simulink model "chain"  (R2022a)
settings: Solver=VariableStepAuto  StartTime=0.0  StopTime=1000  RelTol=1e-3
undefined symbols (not defined in the file): None, S, vsva2197, xcvc1902
libraries: aieBasic x4, aieUtilities x3, dspmlti4 x2, aieDSP x2, hdlUtilities x2, dspsrcs4 x1, vmcUtilities x1, hdlDSPIP x1
settings Model: Creator=abehbood  LastModifiedBy=abehbood
settings ModelReferenceCC: EnableRefExpFcnMdlSchedulingChecks=off
settings RTWCC: Description=Generic Real-Time Target

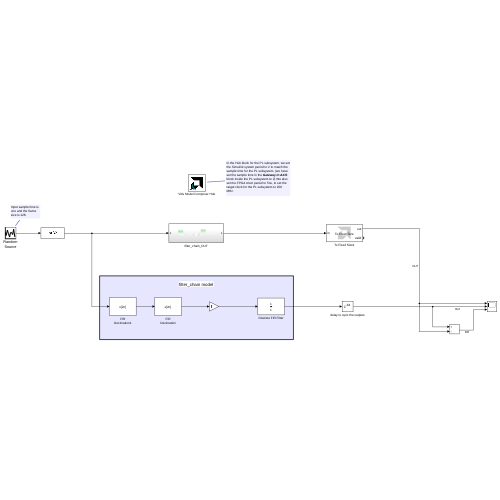
[thumbnail: Simulink's stored preview of the top-level diagram]
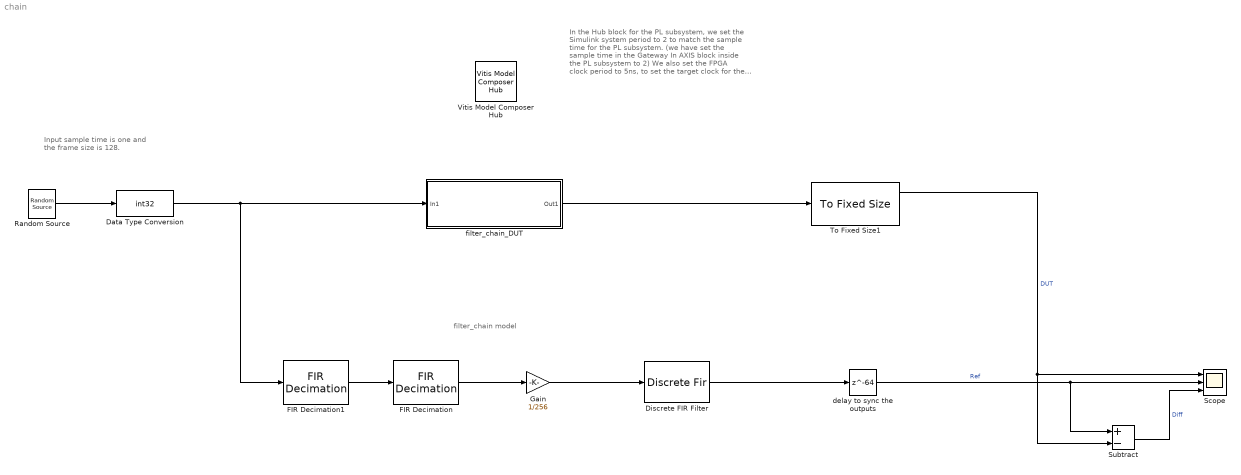
== system chain ==
  note: In the Hub block for the PL subsystem, we set the Simulink system period to 2 to match the sample time for the PL subsystem. (we have set the sample time in the Gateway In AXIS block inside the PL subsystem to 2) We also set the FPGA clock period to 5ns, to set the target clock for the PL subsystem to 200 MHz.
  note: filter_chain model
  note: Input sample time is one and the frame size is 128.
  Data Type Conversion : DataTypeConversion  OutDataTypeStr=int32  SaturateOnIntegerOverflow=off  RndMeth=Floor
  Discrete FIR Filter : DiscreteFir  Coefficients=1  InputProcessing=Columns as channels (frame based)  OutDataTypeStr=Inherit: Same as input
  FIR Decimation : dspmlti4/FIR Decimation  FilterSource=Dialog parameters  h=[6,0,-4,-3,5,6,-6,-13,7,44,64,44,7,-13,-6,6,5,-3,-4,0,6]  D=2  filtStruct=Direct form  FilterObject=FDECIM  InputProcessing=Columns as channels (frame based)  framing=Enforce single-rate processing  inputOffset=0  outputBufInitCond=0  roundingMode=Floor  overflowMode=off  firstCoeffDataTypeStr=Inherit: Same word length as input  firstCoeffMin=[]  firstCoeffMax=[]  firstCoeffLastDataTypeStr=Inherit: Same word length as input  outputMin=[]  outputMax=[]
  FIR Decimation1 : dspmlti4/FIR Decimation  FilterSource=Dialog parameters  h=1  D=2  filtStruct=Direct form  FilterObject=FDECIM  InputProcessing=Columns as channels (frame based)  framing=Enforce single-rate processing  inputOffset=0  outputBufInitCond=0  roundingMode=Floor  overflowMode=off  firstCoeffDataTypeStr=Inherit: Same word length as input  firstCoeffMin=[]  firstCoeffMax=[]  firstCoeffLastDataTypeStr=Inherit: Same word length as input  outputMin=[]  outputMax=[]
  Gain : Gain  Gain=1/256  OutDataTypeStr=Inherit: Same as input
  Random Source : dspsrcs4/Random Source  SrcType=Uniform  NormMethod=Ziggurat  CltLength=12  MinVal=-2^15  MaxVal=2^15-1  MeanVal=0  VarVal=1  RepMode=Not repeatable  rawSeed=1  IsInherit=off  SampMode=Discrete  SampTime=1  SampFrame=128  DataType=Double  OutComplex=Real  OutputFrames=off
  Scope : Scope  NumInputPorts=3
  Subtract : Sum  Inputs=+-
  To Fixed Size1 : aieUtilities/To Fixed Size  Mode=Produce a valid output signal  OutputSize=Inherit: Same as input  CopyMethod=Buffer samples to form output  HasStatusOutput=on
  Vitis Model Composer Hub : vmcUtilities/Vitis Model Composer Hub  Tag=genX  CodeGeneration=off  SubsystemName=filter_chain_DUT  TargetDirectory=./code_hw_emu  ExportType=HW Code  IpVendor=xilinx.com  IpLibrary=hls  IpVersion=1.0  IpHWLanguage=Verilog  AieCompilerOptions={}  AieSimulatorOptions={}  CreateTestbench=off  TestbenchStackSize=10  RunRtlSim=off  RunCSim=off  RunAieSim=on  AieSimTimeout=50000  RunAieSimProfiling=off  LaunchVitisAnalyzer=off  PlotOutput=off  RunX86Sim=off  X86SimTimeout=10  GenHwImage=off  GenLibadfXo=off  PlatformType=Specify Platform  Platform=/proj/xbuilds/SWIP/2024.1_0306_2227/installs/lin64/Vitis/2024.1/base_platforms/xilinx_vck190_base_202410_1/xilinx_vck190_base_202410_1.xpfm  HwSystemType=Baremetal  HwValidationTarget=hw_emu  ProjDevice=Versal VCK190 Evaluation Platform (xcvc1902-vsva2197-2MP-e-S)  ProjDevicePart=xcvc1902-vsva2197-2MP-e-S  AIEType=AIE  SamplePeriod=-1  ClockFrequency=200  DataPathParallelism=1  xilinxfamily=versalaicore  part=xcvc1902  speed=-2MP-e-S  package=vsva2197  directory=./code_hw_emu/ip/PL/src  testbench=on  incr_netlist=off  synthesis_tool=Vivado  clock_wrapper=Clock Enables  dbl_ovrd=According to Block Masks  dcm_input_clock_period=10  sysclk_period=5  simulink_period=2  eval_field=0  IPInfoJsonString="{\"HDLSubsystem\":{\"SubsystemName\":\"PL\",\"IPName\":\"Subsystem\",\"IPLibrary\":\"VMC\",\"IPVendor\":\"User Company\",\"IPVersion\":\"1.0\",\"TargetDirectory\":\"./code_hw_emu\",\"SubsystemDir\":\"./code_hw_emu/ip/PL\"},\"SubsystemTag\":\"DUTNode\",\"AIESubsystem\":{\"SubsystemName\":\"AIE\",\"TargetDirectory\":\"./code_hw_emu\",\"SubsystemDir\":\"./code_hw_emu/ip/AIE\"}}"  LogFileName=/proj/xsjhdstaff4/abehbood/vmc_examples/gitent_ws/Examples/AIENGINE_plus_PL/AIE_HDL/multirate_filter_chain/code_hw_emu/model_composer.log  NThreads=4
  delay to sync the outputs : Delay  DelayLength=64  InputProcessing=Columns as channels (frame based)
  filter_chain_DUT : Subsystem
  wires:
  Random Source/1 -> Data Type Conversion/1
  Data Type Conversion/1 -> FIR Decimation1/1, filter_chain_DUT/1(In1)
  FIR Decimation1/1 -> FIR Decimation/1
  FIR Decimation/1 -> Gain/1
  To Fixed Size1/1 -> Subtract/2, Scope/1  "DUT"
  Gain/1 -> Discrete FIR Filter/1
  Subtract/1 -> Scope/3  "Diff"
  Discrete FIR Filter/1 -> delay to sync the outputs/1
  filter_chain_DUT/1(Out1) -> To Fixed Size1/1
  delay to sync the outputs/1 -> Subtract/1, Scope/2  "Ref"

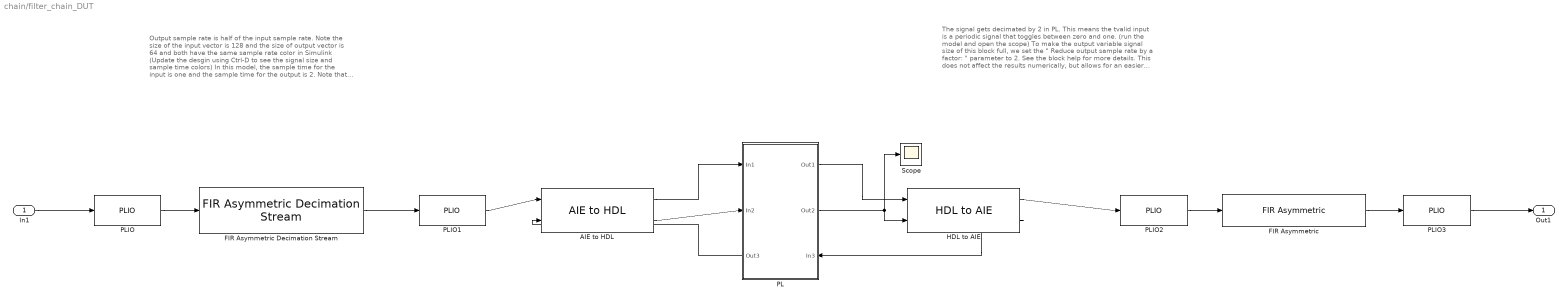
== system chain/filter_chain_DUT ==
  note: Output sample rate is half of the input sample rate. Note the size of the input vector is 128 and the size of output vector is 64 and both have the same sample rate color in Simulink (Update the desgin using Ctrl-D to see the signal size and sample time colors)
      |
      | In this model, the sample time for the input is one and the sample time for the output is 2. Note that the Simulink Timing Legend shows the period for the frames. For example the period of the signal in green is 128. Since the size of the input signal is also 128, this signal has a sample time of 1.
  note: The signal gets decimated by 2 in PL. This means the tvalid input is a periodic signal that toggles between zero and one. (run the model and open the scope)
      |
      | To make the output variable signal size of this block full, we set the " Reduce output sample rate by a factor: " parameter to 2. See the block help for more details. This does not affect the results numerically, but allows for an easier monitoring and visualization of the signals.
      |
      | To learn more about variable size signals click here.
  In1 : Inport
  AIE to HDL : aieUtilities/AIE to HDL  OutDataType=int32  OutSampleTime=Inherit: Same as tready
  FIR Asymmetric : aieDSP/FIR Asymmetric  data_type=int32  coef_type=int16  use_coeff_reload=off  num_outputs=off  coeff=[1, zeros(1,31)]  fir_length=32  input_window_size=32  shift_val=0  rnd_mode=Floor  sat_mode=0-None  casc_length=1  blockJsonConstraints=[]  blockJsonConstraintsInternal=[]  spec=vmc_fir_sr_asym.json  SerializedMaskParamNames=[]  SerializedMaskParamValues=[]  SerializedMaskParamVisibilities=[]  block_type=FIR Asymmetric  SerializedMaskParamDataypes=typename|typename|bool|bool|coef_type|uint|uint|uint|uint|uint|uint|uint  SerializedMaskParamEnumStrArr=0|0|0|0|0|0|0|0|Floor,Ceiling,Round to positive infinity,Round to negative infinity,Round symmetrical to infinity,Round symmetrical to zero,Round convergent to even,Round convergent to odd|0-None,1-Asymmetric,3-Symmetric|0|0  SerializedMaskParamEnumValArr=0|0|0|0|0|0|0|0|0,1,2,3,4,5,6,7|0,1,3|0|0  SerializedMaskParamVectorArr=0|0|0|0|1|0|0|0|0|0|0|0
  FIR Asymmetric Decimation Stream : aieDSP/FIR Asymmetric Decimation Stream  data_type=int32  coef_type=int16  use_coeff_reload=off  dual_ip=off  num_outputs=off  coeff=[1, zeros(1,25)]  fir_length=26  decimate_factor=2  input_window_size=128  shift_val=0  rnd_mode=Floor  sat_mode=0-None  ssr=1  deci_poly=1  casc_length=4  blockJsonConstraints=[]  blockJsonConstraintsInternal=[]  spec=vmc_stream_fir_decimate_asym.json  SerializedMaskParamNames=[]  SerializedMaskParamValues=[]  SerializedMaskParamVisibilities=[]  block_type=FIR Asymmetric Decimation Stream  SerializedMaskParamDataypes=typename|typename|bool|bool|bool|coef_type|uint|uint|uint|uint|uint|uint|uint|uint|uint|uint  SerializedMaskParamEnumStrArr=0|0|0|0|0|0|0|0|0|0|Floor,Ceiling,Round to positive infinity,Round to negative infinity,Round symmetrical to infinity,Round symmetrical to zero,Round convergent to even,Round convergent to odd|0-None,1-Asymmetric,3-Symmetric|0|0|0|0  SerializedMaskParamEnumValArr=0|0|0|0|0|0|0|0|0|0|0,1,2,3,4,5,6,7|0,1,3|0|0|0|0  SerializedMaskParamVectorArr=0|0|0|0|0|1|0|0|0|0|0|0|0|0|0|0
  HDL to AIE : aieUtilities/HDL to AIE  InDataType=int32  OutDataType=int32  OutSampleTime=16  SamplesPerFrame=32  RateReduceFactor=2  ManuallySpecifyOutSampleTime=off
  PL : Subsystem
      settings: PortSchema="{\"entries\":[{\"content\":{\"sides\":[{\"content\":{\"connectorIds\":[\"In1\",\"In2\",\"Out3\"]},\"type\":\"ConnectorPlacement.EquallySpacedRectSide\",\"uuid\":\"b9240e68-8c33-49ba-b00e-74953cef8815\"},{\"content\":{\"connectorIds\":[\"Out1\",\"Out2\",\"In3\"],\"side\":\"RIGHT\"},\"type\":\"ConnectorPlacement.EquallySpacedRectSide\",\"uuid\":\"ae9f69ab-13df-4ed6-8e03-b2ffeca92de6\"},{\"content\":{\"side\":\"TOP\"},\"type\":\"ConnectorPlacement.EquallySpacedRectSide\",\"uuid\":\"62802255-d0c0-4e5e-87ba-02035ab73d0f\"}]},\"type\":\"ConnectorPlacement.EquallySpacedConnector\",\"uuid\":\"85ea88ef-d819-4f47-a821-adcbfe47cef7\"}],\"packageUris\":[\"http://schema.mathworks.com/mf0/Connector/R2020b\"],\"version\":\"1.0\"}"
  PLIO : aieBasic/PLIO  PlioWidth=64  PlioFreqSpec=on  PlioFreq=400  ColLocation=0  channel=0  blockJsonConstraints=[]  deprecateConstraints=0
  PLIO1 : aieBasic/PLIO  PlioWidth=32  PlioFreqSpec=off  PlioFreq=250  ColLocation=0  channel=0  blockJsonConstraints=[]  deprecateConstraints=0
  PLIO2 : aieBasic/PLIO  PlioWidth=32  PlioFreqSpec=on  PlioFreq=400  ColLocation=0  channel=0  blockJsonConstraints=[]  deprecateConstraints=0
  PLIO3 : aieBasic/PLIO  PlioWidth=32  PlioFreqSpec=off  PlioFreq=250  ColLocation=0  channel=0  blockJsonConstraints=[]  deprecateConstraints=0
  Scope : Scope
  Out1 : Outport
  wires:
  PL/3(Out3) -> AIE to HDL/2
  AIE to HDL/1 -> PL/1(In1)
  PL/2(Out2) -> Scope/1, HDL to AIE/2
  HDL to AIE/2 -> PL/3(In3)
  PLIO1/1 -> AIE to HDL/1
  PLIO3/1 -> Out1/1
  PL/1(Out1) -> HDL to AIE/1
  AIE to HDL/2 -> PL/2(In2)
  FIR Asymmetric/1 -> PLIO3/1
  In1/1 -> PLIO/1
  HDL to AIE/1 -> PLIO2/1
  PLIO/1 -> FIR Asymmetric Decimation Stream/1
  PLIO2/1 -> FIR Asymmetric/1
  FIR Asymmetric Decimation Stream/1 -> PLIO1/1

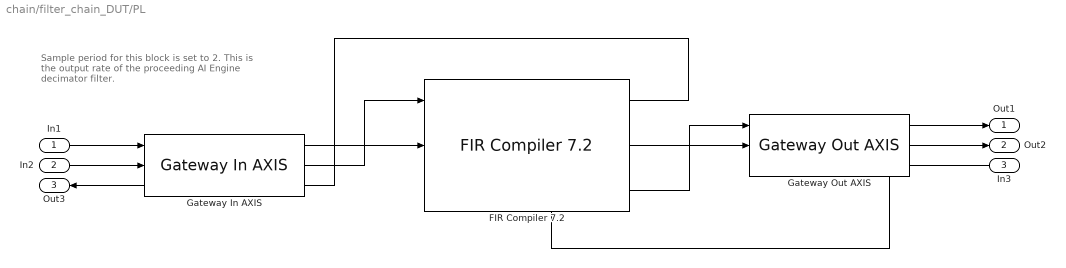
== system chain/filter_chain_DUT/PL ==
  note: Sample period for this block is set to 2. This is the output rate of the proceeding AI Engine decimator filter.
  In1 : Inport
  In2 : Inport  Port=2
  In3 : Inport  Port=3
  FIR Compiler 7.2 : hdlDSPIP/FIR Compiler 7.2   coefficientvector=[6,0,-4,-3,5,6,-6,-13,7,44,64,44,7,-13,-6,6,5,-3,-4,0,6]  coefficient_sets=1  coefficient_reload=off  filter_type=Decimation  rate_change_type=Integer  interpolation_rate=1  decimation_rate=2  zero_pack_factor=1  channel_sequence=Basic  number_channels=1  pattern_list='P4-0,P4-1,P4-2,P4-3,P4-4'  number_paths=1  ratespecification=Input_Sample_Period  sampleperiod=1  hardwareoversamplingrate=1  coefficient_sign=Signed  quantization=Integer_Coefficients  coefficient_width=16  bestprecision=off  coefficient_fractional_bits=0  coefficient_structure=Inferred  output_rounding_mode=Truncate_LSBs  output_width=32  filter_architecture=Systolic_Multiply_Accumulate  optimization_goal=Area  optimization_list='None'  data_buffer_type=Automatic  coefficient_buffer_type=Automatic  input_buffer_type=Automatic  output_buffer_type=Automatic  preference_for_other_storage=Automatic  multi_column_support=Automatic  columnconfig='3'  inter_column_pipe_length=4  data_has_tlast=Not_Required  m_data_has_tready=on  s_data_has_fifo=on  s_data_has_tuser=Not_Required  m_data_has_tuser=Not_Required  s_config_sync_mode=On_Vector  s_config_method=Single  num_reload_slots=1  has_aclken=off  has_aresetn=off  reset_data_vector=on  trim_axipin_name=on  simulation_type=hybrid_sim  simulation_model=sysgen:xfirv7_2_cmodel  data_path_portlist={ 's_axis_data_tdata', 'm_axis_data_tdata' }  passband_min=0.0  passband_max=0.5  stopband_min=0.5  stopband_max=1.0  filter_selection=1  gui_behaviour='Sysgen_GUI'  data_sign=Signed  data_width=16  data_fractional_bits=0  data_tuser_width=1  wrapper_available=true  ip_wrap_arbitrary_binary_point=true  ip_name=FIR Compiler  ip_version=7.2  dsptool_ready=true  ipcore_usecache=true  ipcore_useipmodelcache=true  port_translation_map={ 'aclken' => 'en', 'aresetn' => 'rst' }  run_core_at_system_period=true  ipcore_xco_need_fpga_part=true  ipcore_fpga_part=[]  XmcBlockStatus=1  maskContainerNames=tabcontainer1  block_type=fir_compiler_v7_2  block_config=sysgen:rodinimport_config  block_width=820  block_height=600
  Gateway In AXIS : hdlUtilities/Gateway In AXIS  gui_display_data_type=Fixed-point  arith_type=Signed (2's comp)  n_bits=32  bin_pt=0  preci_type=Custom  exp_width=16  frac_width=24  quantization=Truncate  overflow=Flag as error  OutSampleTime=2  block_type=gatewayinaxi  XmcBlockStatus=1
  Gateway Out AXIS : hdlUtilities/Gateway Out AXIS  mask_sample_period=2  block_type=gatewayoutaxi
  Out1 : Outport
  Out2 : Outport  Port=2
  Out3 : Outport  Port=3
  wires:
  Gateway Out AXIS/2 -> Out2/1
  In2/1 -> Gateway In AXIS/2
  FIR Compiler 7.2/3 -> Gateway Out AXIS/1
  Gateway Out AXIS/3 -> FIR Compiler 7.2/3
  Gateway In AXIS/2 -> FIR Compiler 7.2/1
  Gateway In AXIS/1 -> FIR Compiler 7.2/2
  Gateway In AXIS/3 -> Out3/1
  In3/1 -> Gateway Out AXIS/3
  Gateway Out AXIS/1 -> Out1/1
  FIR Compiler 7.2/2 -> Gateway Out AXIS/2
  FIR Compiler 7.2/1 -> Gateway In AXIS/3
  In1/1 -> Gateway In AXIS/1
